simulink model "test1"  (R2022b)
settings: Solver=VariableStepAuto  StartTime=0.0  StopTime=120  RelTol=1e-3
libraries: simulink x7, simulink_extras x3, slpidlib x1
settings Model: Creator=littl  LastModifiedBy=littl

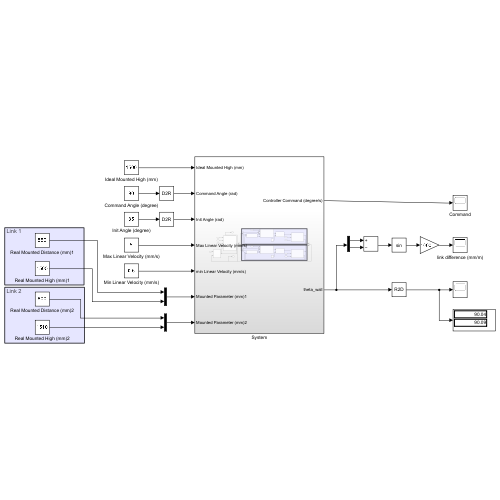
[thumbnail: Simulink's stored preview of the top-level diagram]
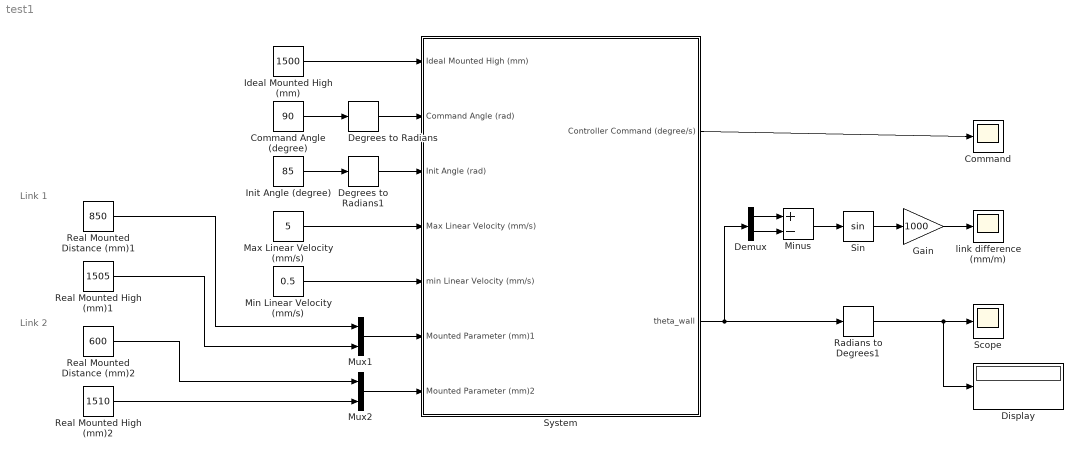
== system test1 ==
  note: Link 1
  note: Link 2
  Command : Scope
  Command Angle (degree) : Constant  Value=90
  Degrees to Radians : simulink_extras/Transformations/Degrees to Radians
  Degrees to Radians1 : simulink_extras/Transformations/Degrees to Radians
  Demux : Demux  Outputs=2
  Display : Display
  Gain : Gain  Gain=1000
  Ideal Mounted High (mm) : Constant  Value=1500
  Init Angle (degree) : Constant  Value=85
  Max Linear Velocity (mm/s) : Constant  Value=5
  Min Linear Velocity (mm/s) : Constant  Value=0.5
  Minus : Sum  Inputs=+-
  Mux1 : Mux  Inputs=2
  Mux2 : Mux  Inputs=2
  Radians to Degrees1 : simulink_extras/Transformations/Radians to Degrees
  Real Mounted Distance (mm)1 : Constant  Value=850
  Real Mounted Distance (mm)2 : Constant  Value=600
  Real Mounted High (mm)1 : Constant  Value=1505
  Real Mounted High (mm)2 : Constant  Value=1510
  Scope : Scope
  Sin : Trigonometry
  System : Subsystem
  link difference (mm/m) : Scope
  wires:
  Command Angle (degree)/1 -> Degrees to Radians/1
  Init Angle (degree)/1 -> Degrees to Radians1/1
  Minus/1 -> Sin/1
  Ideal Mounted High (mm)/1 -> System/1(Ideal Mounted High (mm))
  Degrees to Radians/1 -> System/2(Command Angle (rad))
  Degrees to Radians1/1 -> System/3(Init Angle (rad))
  System/1(Controller Command (degree/s)) -> Command/1
  Max Linear Velocity (mm/s)/1 -> System/4(Max Linear Velocity (mm/s))
  Min Linear Velocity (mm/s)/1 -> System/5(min Linear Velocity (mm/s))
  Demux/2 -> Minus/2
  Demux/1 -> Minus/1
  Radians to Degrees1/1 -> Display/1, Scope/1
  Sin/1 -> Gain/1
  Gain/1 -> link difference (mm/m)/1
  System/2(theta_wall) -> Radians to Degrees1/1, Demux/1
  Mux1/1 -> System/6(Mounted Parameter (mm)1)
  Real Mounted Distance (mm)1/1 -> Mux1/1
  Real Mounted High (mm)1/1 -> Mux1/2
  Real Mounted Distance (mm)2/1 -> Mux2/1
  Real Mounted High (mm)2/1 -> Mux2/2
  Mux2/1 -> System/7(Mounted Parameter (mm)2)

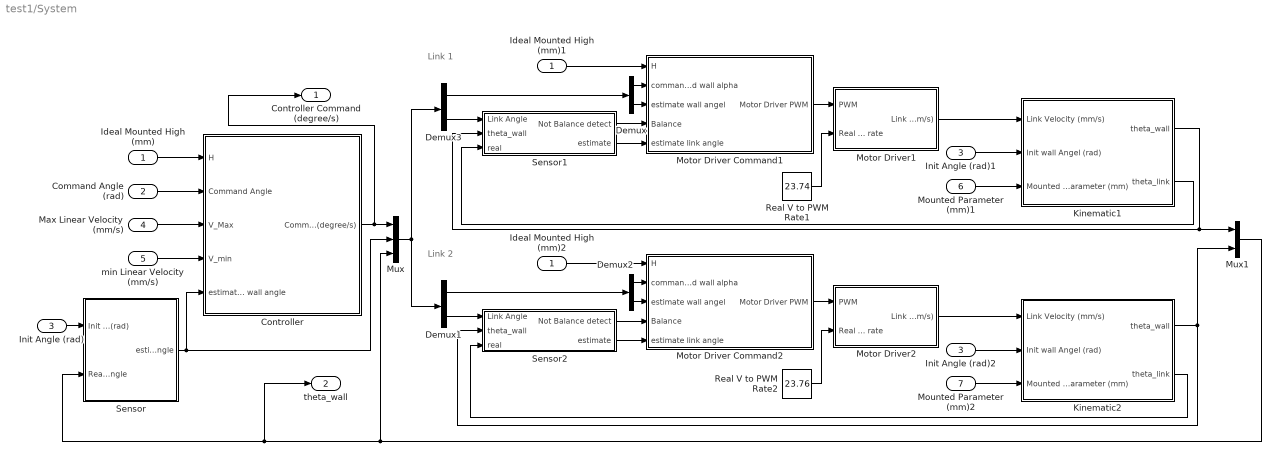
== system test1/System ==
  note: Link 1
  note: Link 2
  Ideal Mounted High (mm) : Inport
  Command Angle (rad) : Inport  Port=2
  Init Angle (rad) : Inport  Port=3
  Max Linear Velocity (mm/s) : Inport  Port=4
  min Linear Velocity (mm/s) : Inport  Port=5
  Mounted Parameter (mm)1 : Inport  Port=6
  Mounted Parameter (mm)2 : Inport  Port=7
  Controller : Subsystem
  Demux{,1..3} (4 alike) : Demux  Outputs=2
  Ideal Mounted High (mm)1 : InportShadow
  Ideal Mounted High (mm)2 : InportShadow
  Init Angle (rad)1 : InportShadow  Port=3
  Init Angle (rad)2 : InportShadow  Port=3
  Kinematic1 : Subsystem
  Kinematic2 : Subsystem
  Motor Driver Command1 : Subsystem
  Motor Driver Command2 : Subsystem
  Motor Driver1 : Subsystem
  Motor Driver2 : Subsystem
  Mux : Mux  Inputs=3
  Mux1 : Mux  Inputs=2
  Real V to PWM Rate1 : Constant  Value=23.74
  Real V to PWM Rate2 : Constant  Value=23.76
  Sensor : Subsystem
  Sensor1 : Subsystem
  Sensor2 : Subsystem
  Controller Command (degree/s) : Outport
  theta_wall : Outport  Port=2
  wires:
  min Linear Velocity (mm/s)/1 -> Controller/4(V_min)
  Motor Driver Command2/1(Motor Driver PWM) -> Motor Driver2/1(PWM)
  Real V to PWM Rate1/1 -> Motor Driver1/2(Real V to PWM rate)
  Max Linear Velocity (mm/s)/1 -> Controller/3(V_Max)
  Kinematic2/1(theta_wall) -> Mux1/2, Sensor2/2(theta_wall)
  Command Angle (rad)/1 -> Controller/2(Command Angle)
  Mounted Parameter (mm)2/1 -> Kinematic2/3(Mounted Parameter (mm))
  Real V to PWM Rate2/1 -> Motor Driver2/2(Real V to PWM rate)
  Controller/1(Command alpha (degree/s)) -> Controller Command (degree/s)/1, Mux/1
  Mounted Parameter (mm)1/1 -> Kinematic1/3(Mounted Parameter (mm))
  Motor Driver Command1/1(Motor Driver PWM) -> Motor Driver1/1(PWM)
  Motor Driver1/1(Link Velocity (mm/s)) -> Kinematic1/1(Link Velocity (mm/s))
  Motor Driver2/1(Link Velocity (mm/s)) -> Kinematic2/1(Link Velocity (mm/s))
  Ideal Mounted High (mm)2/1 -> Motor Driver Command2/1(H)
  Ideal Mounted High (mm)/1 -> Controller/1(H)
  Init Angle (rad)1/1 -> Kinematic1/2(Init wall Angel (rad))
  Init Angle (rad)2/1 -> Kinematic2/2(Init wall Angel (rad))
  Mux/1 -> Demux3/1, Demux1/1
  Sensor/1(estimate wall angle) -> Controller/5(estimate wall angle), Mux/2
  Init Angle (rad)/1 -> Sensor/1(Init Angle (rad))
  Kinematic1/1(theta_wall) -> Mux1/1, Sensor1/2(theta_wall)
  Mux1/1 -> Mux/3, theta_wall/1, Sensor/2(Real Angle)
  Demux2/1 -> Motor Driver Command2/2(command wall alpha)
  Demux2/2 -> Motor Driver Command2/3(estimate wall angel)
  Demux1/1 -> Demux2/1
  Demux/1 -> Motor Driver Command1/2(command wall alpha)
  Demux/2 -> Motor Driver Command1/3(estimate wall angel)
  Ideal Mounted High (mm)1/1 -> Motor Driver Command1/1(H)
  Demux3/1 -> Demux/1
  Demux3/2 -> Sensor1/1(Link Angle)
  Kinematic1/2(theta_link) -> Sensor1/3(real)
  Sensor1/1(Not Balance detect) -> Motor Driver Command1/4(Balance)
  Sensor1/2(estimate) -> Motor Driver Command1/5(estimate link angle)
  Demux1/2 -> Sensor2/1(Link Angle)
  Kinematic2/2(theta_link) -> Sensor2/3(real)
  Sensor2/1(Not Balance detect) -> Motor Driver Command2/4(Balance)
  Sensor2/2(estimate) -> Motor Driver Command2/5(estimate link angle)

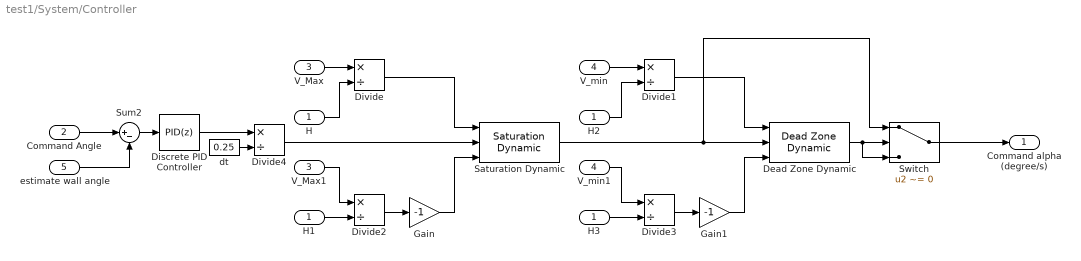
== system test1/System/Controller ==
  H : Inport
  Command Angle : Inport  Port=2
  V_Max : Inport  Port=3
  V_min : Inport  Port=4
  estimate wall angle : Inport  Port=5
  Dead Zone Dynamic : simulink/Discontinuities/Dead Zone Dynamic
  Discrete PID Controller : slpidlib/PID Controller  Controller=PID  Form=Parallel  TimeDomain=Discrete-time  UseExternalTs=off  SampleTime=0.25  IntegratorMethod=Forward Euler  FilterMethod=Forward Euler  ControllerParametersSource=internal  P=0.13  I=3e-5  UseKiTs=off  D=0.1  N=100  UseFilter=off  TunerSelectOption=Transfer Function Based (PID Tuner App)  ZeroCross=off  InitialConditionSource=internal  InitialConditionForIntegrator=0  InitialConditionForFilter=0  DifferentiatorICPrevScaledInput=0  ExternalReset=none  TrackingMode=off  Kt=1  LimitOutput=off  SatLimitsSource=internal  UpperSaturationLimit=inf  LowerSaturationLimit=-inf  LinearizeAsGain=off  AntiWindupMode=none  Kb=1  LimitIntegrator=off  UpperIntegratorSaturationLimit=inf  LowerIntegratorSaturationLimit=-inf  RndMeth=Ceiling  PGainOutDataTypeStr=Inherit: Inherit via back propagation  PProdOutDataTypeStr=Inherit: Inherit via back propagation  POutMin=[]  POutMax=[]  IOutMin=[]  IOutMax=[]  DOutMin=[]  DOutMax=[]  NOutMin=[]  NOutMax=[]  SumOutMin=[]  SumOutMax=[]  SaturationOutMin=[]  SaturationOutMax=[]  PParamMin=[]  PParamMax=[]  IParamMin=[]  IParamMax=[]  DParamMin=[]  DParamMax=[]  NParamMin=[]  NParamMax=[]  KbParamMin=[]  KbParamMax=[]  KtParamMin=[]  KtParamMax=[]  KbOutMin=[]  KbOutMax=[]  KtOutMin=[]  KtOutMax=[]  IntegratorOutMin=[]  IntegratorOutMax=[]  FilterOutMin=[]  FilterOutMax=[]  SumI1OutMin=[]  SumI1OutMax=[]  SumI2OutMin=[]  SumI2OutMax=[]  SumI3OutMin=[]  SumI3OutMax=[]  SumI4OutMin=[]  SumI4OutMax=[]  SumDOutMin=[]  SumDOutMax=[]  DifferentiatorOutMin=[]  DifferentiatorOutMax=[]  FilterDiffOutCoefMin=[]  FilterDiffOutCoefMax=[]  ReciprocalOutMin=[]  ReciprocalOutMax=[]  SumDenOutMin=[]  SumDenOutMax=[]  SumNumOutMin=[]  SumNumOutMax=[]  DivideOutMin=[]  DivideOutMax=[]  UdiffTsProdOutMin=[]  UdiffTsProdOutMax=[]  NTsProdOutMin=[]  NTsProdOutMax=[]  UintegralTsProdOutMin=[]  UintegralTsProdOutMax=[]  UngainTsProdOutMin=[]  UngainTsProdOutMax=[]  ClampingZeroOutDataTypeStr=Inherit: Inherit via back propagation  ClampingZeroOutMin=[]  ClampingZeroOutMax=[]  FilterDenConstantOutDataTypeStr=Inherit: Inherit via back propagation  FilterDenConstantOutMin=[]  FilterDenConstantOutMax=[]  PCopyOutDataTypeStr=Inherit: Inherit via back propagation  PCopyOutMin=[]  PCopyOutMax=[]  NCopyOutDataTypeStr=Inherit: Inherit via back propagation  NCopyOutMin=[]  NCopyOutMax=[]  IntegratorContinuousStateAttributes=''  IntegratorStateMustResolveToSignalObject=off  IntegratorRTWStateStorageClass=Auto  FilterContinuousStateAttributes=''  FilterStateMustResolveToSignalObject=off  FilterRTWStateStorageClass=Auto  ParallelPVariant=InternalParameters  IdealPVariant=Disabled  IVariant=InternalParameters  DVariant=InternalParameters  IntegratorVariant=Discrete  SatVariant=Disabled  AWVariant=Passthrough  PCopyVariant=Disabled  TRVariant=Disabled  FdbkBlocksVariant=Forward  IdealPFdbkVariant=Disabled  SatFdbkVariant=Disabled  DerivativeFilterVariant=Differentiator  NVariant=Passthrough  NCopyVariant=Disabled_SignalSpec  FilterICVariant=InternalICsDifferentiator  IntegratorICVariant=InternalICs  ExternalResetVariant=Disabled  TRSumVariant=Passthrough  SumFdbkVariant=Disabled  SumVariant=Sum_PID  TsampFilterVariant=InternalTs  TsampNgainVariant=Passthrough  TsampIntegralVariant=Passthrough  ExternalSaturationOutDataTypeStr=Inherit: Same as second input
      settings: LibrarySourceBlock=simulink/Discrete/Discrete PID Controller
  Divide{,1..4} (5 alike) : Product  Inputs=*/
  Gain : Gain  Gain=-1
  Gain1 : Gain  Gain=-1
  H1 : InportShadow
  H2 : InportShadow
  H3 : InportShadow
  Saturation Dynamic : simulink/Discontinuities/Saturation Dynamic  OutMin=[]  OutMax=[]  OutDataTypeStr=Inherit: Same as second input  OutDataType=fixdt(1, 16)  OutScaling=2^-10  DoSatur=off
  Sum2 : Sum  Inputs=|+-
  Switch : Switch  Criteria=u2 ~= 0  SaturateOnIntegerOverflow=off  InputSameDT=off
  V_Max1 : InportShadow  Port=3
  V_min1 : InportShadow  Port=4
  dt : Constant  Value=0.25
  Command alpha (degree/s) : Outport
  wires:
  Sum2/1 -> Discrete PID Controller/1
  Command Angle/1 -> Sum2/1
  estimate wall angle/1 -> Sum2/2
  Divide2/1 -> Gain/1
  H1/1 -> Divide2/2
  V_Max/1 -> Divide/1
  H/1 -> Divide/2
  Gain/1 -> Saturation Dynamic/3
  Divide/1 -> Saturation Dynamic/1
  H3/1 -> Divide3/2
  V_min1/1 -> Divide3/1
  H2/1 -> Divide1/2
  V_min/1 -> Divide1/1
  Divide1/1 -> Dead Zone Dynamic/1
  Divide3/1 -> Gain1/1
  Gain1/1 -> Dead Zone Dynamic/3
  V_Max1/1 -> Divide2/1
  Saturation Dynamic/1 -> Switch/1, Dead Zone Dynamic/2
  Dead Zone Dynamic/1 -> Switch/3, Switch/2
  Switch/1 -> Command alpha (degree/s)/1
  Discrete PID Controller/1 -> Divide4/1
  Divide4/1 -> Saturation Dynamic/2
  dt/1 -> Divide4/2

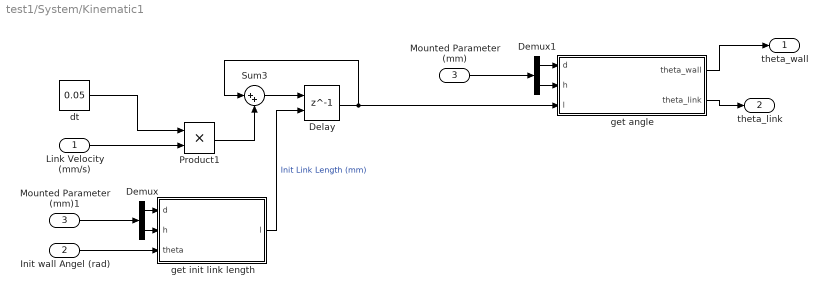
== system test1/System/Kinematic1 ==
  Link Velocity (mm/s) : Inport
  Init wall Angel (rad) : Inport  Port=2
  Mounted Parameter (mm) : Inport  Port=3
  Delay : Delay  DelayLength=1  InitialConditionSource=Input port  SampleTime=0.125
      settings: InputPortMap=u0,p4
  Demux : Demux  Outputs=2
  Demux1 : Demux  Outputs=2
  Mounted Parameter (mm)1 : InportShadow  Port=3
  Product1 : Product
  Sum3 : Sum  Inputs=|++
  dt : Constant  Value=0.05
  get angle : MATLAB Function  TreatAsAtomicUnit=on
  get init link length : MATLAB Function  TreatAsAtomicUnit=on
  theta_wall : Outport
  theta_link : Outport  Port=2
  wires:
  get angle/2(theta_link) -> theta_link/1
  get angle/1(theta_wall) -> theta_wall/1
  Sum3/1 -> Delay/1
  Delay/1 -> Sum3/1, get angle/3(l)
  Product1/1 -> Sum3/2
  get init link length/1(l) -> Delay/2  "Init Link Length (mm)"
  Init wall Angel (rad)/1 -> get init link length/3(theta)
  Link Velocity (mm/s)/1 -> Product1/2
  dt/1 -> Product1/1
  Demux/1 -> get init link length/1(d)
  Mounted Parameter (mm)1/1 -> Demux/1
  Demux/2 -> get init link length/2(h)
  Demux1/1 -> get angle/1(d)
  Demux1/2 -> get angle/2(h)
  Mounted Parameter (mm)/1 -> Demux1/1

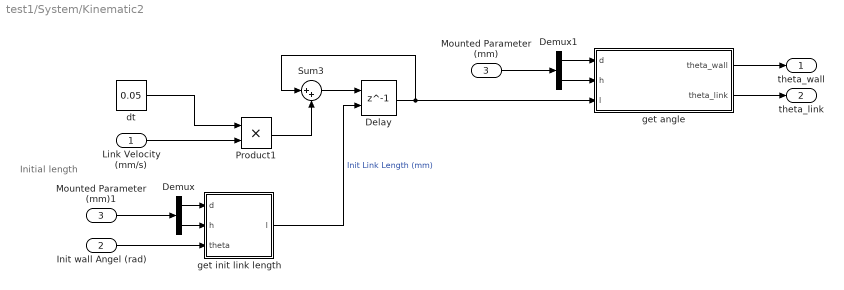
== system test1/System/Kinematic2 ==
  note: Initial length
  Link Velocity (mm/s) : Inport
  Init wall Angel (rad) : Inport  Port=2
  Mounted Parameter (mm) : Inport  Port=3
  Delay : Delay  DelayLength=1  InitialConditionSource=Input port  SampleTime=0.125
      settings: InputPortMap=u0,p4
  Demux : Demux  Outputs=2
  Demux1 : Demux  Outputs=2
  Mounted Parameter (mm)1 : InportShadow  Port=3
  Product1 : Product
  Sum3 : Sum  Inputs=|++
  dt : Constant  Value=0.05
  get angle : MATLAB Function  TreatAsAtomicUnit=on
  get init link length : MATLAB Function  TreatAsAtomicUnit=on
  theta_wall : Outport
  theta_link : Outport  Port=2
  wires:
  get angle/2(theta_link) -> theta_link/1
  get angle/1(theta_wall) -> theta_wall/1
  Sum3/1 -> Delay/1
  Delay/1 -> Sum3/1, get angle/3(l)
  Product1/1 -> Sum3/2
  get init link length/1(l) -> Delay/2  "Init Link Length (mm)"
  Init wall Angel (rad)/1 -> get init link length/3(theta)
  Link Velocity (mm/s)/1 -> Product1/2
  dt/1 -> Product1/1
  Demux/1 -> get init link length/1(d)
  Demux/2 -> get init link length/2(h)
  Mounted Parameter (mm)1/1 -> Demux/1
  Mounted Parameter (mm)/1 -> Demux1/1
  Demux1/1 -> get angle/1(d)
  Demux1/2 -> get angle/2(h)

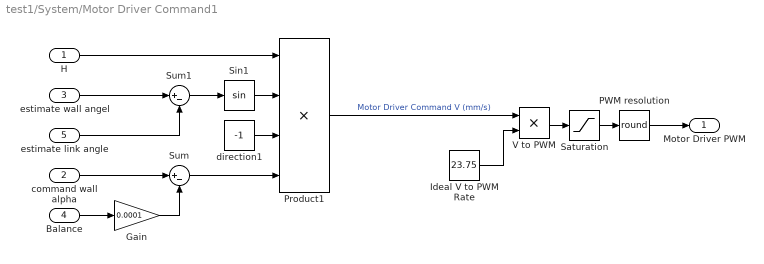
== system test1/System/Motor Driver Command1 ==
  H : Inport
  command wall alpha : Inport  Port=2
  estimate wall angel : Inport  Port=3
  Balance : Inport  Port=4
  estimate link angle : Inport  Port=5
  Gain : Gain  Gain=0.0001
  Ideal V to PWM Rate : Constant  Value=23.75
  PWM resolution : Rounding  Operator=round
  Product1 : Product  Inputs=4
  Saturation : Saturate  UpperLimit=255  LowerLimit=-255
  Sin1 : Trigonometry
  Sum : Sum  Inputs=|+-
  Sum1 : Sum  Inputs=|+-
  V to PWM : Product
  direction1 : Constant  Value=-1
  Motor Driver PWM : Outport
  wires:
  Ideal V to PWM Rate/1 -> V to PWM/2
  V to PWM/1 -> Saturation/1
  Saturation/1 -> PWM resolution/1
  PWM resolution/1 -> Motor Driver PWM/1
  Balance/1 -> Gain/1
  Sin1/1 -> Product1/2
  estimate link angle/1 -> Sum1/2
  Gain/1 -> Sum/2
  command wall alpha/1 -> Sum/1
  estimate wall angel/1 -> Sum1/1
  H/1 -> Product1/1
  Sum/1 -> Product1/4
  direction1/1 -> Product1/3
  Sum1/1 -> Sin1/1
  Product1/1 -> V to PWM/1  "Motor Driver Command V (mm/s)"

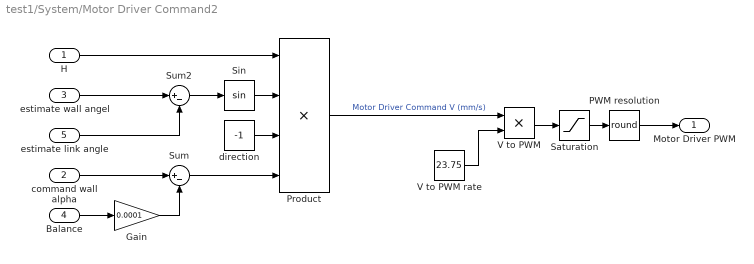
== system test1/System/Motor Driver Command2 ==
  H : Inport
  command wall alpha : Inport  Port=2
  estimate wall angel : Inport  Port=3
  Balance : Inport  Port=4
  estimate link angle : Inport  Port=5
  Gain : Gain  Gain=0.0001
  PWM resolution : Rounding  Operator=round
  Product : Product  Inputs=4
  Saturation : Saturate  UpperLimit=255  LowerLimit=-255
  Sin : Trigonometry
  Sum : Sum  Inputs=|+-
  Sum2 : Sum  Inputs=|+-
  V to PWM : Product
  V to PWM rate : Constant  Value=23.75
  direction : Constant  Value=-1
  Motor Driver PWM : Outport
  wires:
  Sum2/1 -> Sin/1
  estimate link angle/1 -> Sum2/2
  Saturation/1 -> PWM resolution/1
  Product/1 -> V to PWM/1  "Motor Driver Command V (mm/s)"
  V to PWM rate/1 -> V to PWM/2
  PWM resolution/1 -> Motor Driver PWM/1
  V to PWM/1 -> Saturation/1
  estimate wall angel/1 -> Sum2/1
  Balance/1 -> Gain/1
  command wall alpha/1 -> Sum/1
  Gain/1 -> Sum/2
  H/1 -> Product/1
  Sin/1 -> Product/2
  direction/1 -> Product/3
  Sum/1 -> Product/4

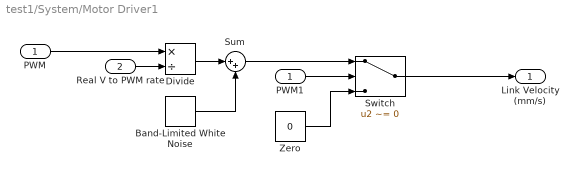
== system test1/System/Motor Driver1 ==
  PWM : Inport
  Real V to PWM rate : Inport  Port=2
  Band-Limited White Noise : simulink/Sources/Band-Limited White Noise  Cov=[0.001]  Ts=0.05  seed=[23341]
  Divide : Product  Inputs=*/
  PWM1 : InportShadow
  Sum : Sum  Inputs=|++
  Switch : Switch  Criteria=u2 ~= 0  SaturateOnIntegerOverflow=off  InputSameDT=off
  Zero : Constant  Value=0  OutDataTypeStr=Inherit: Inherit via back propagation
  Link Velocity (mm/s) : Outport
  wires:
  Switch/1 -> Link Velocity (mm/s)/1
  Real V to PWM rate/1 -> Divide/2
  PWM/1 -> Divide/1
  Divide/1 -> Sum/1
  Band-Limited White Noise/1 -> Sum/2
  Sum/1 -> Switch/1
  PWM1/1 -> Switch/2
  Zero/1 -> Switch/3

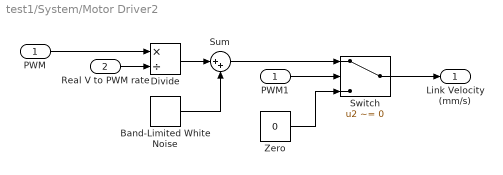
== system test1/System/Motor Driver2 ==
  PWM : Inport
  Real V to PWM rate : Inport  Port=2
  Band-Limited White Noise : simulink/Sources/Band-Limited White Noise  Cov=[0.001]  Ts=0.05  seed=[23341]
  Divide : Product  Inputs=*/
  PWM1 : InportShadow
  Sum : Sum  Inputs=|++
  Switch : Switch  Criteria=u2 ~= 0  SaturateOnIntegerOverflow=off  InputSameDT=off
  Zero : Constant  Value=0  OutDataTypeStr=Inherit: Inherit via back propagation
  Link Velocity (mm/s) : Outport
  wires:
  Switch/1 -> Link Velocity (mm/s)/1
  Real V to PWM rate/1 -> Divide/2
  PWM/1 -> Divide/1
  Divide/1 -> Sum/1
  Band-Limited White Noise/1 -> Sum/2
  Sum/1 -> Switch/1
  PWM1/1 -> Switch/2
  Zero/1 -> Switch/3

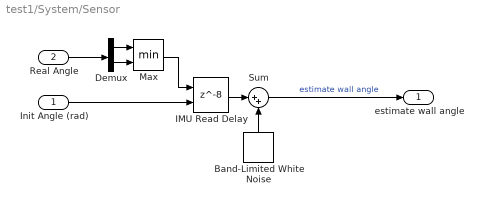
== system test1/System/Sensor ==
  Init Angle (rad) : Inport
  Real Angle : Inport  Port=2
  Band-Limited White Noise : simulink/Sources/Band-Limited White Noise  Cov=1e-10  Ts=0.05  seed=[23341]
  Demux : Demux  Outputs=2
  IMU Read Delay : Delay  DelayLength=8  InitialConditionSource=Input port  SampleTime=0.25
      settings: InputPortMap=u0,p4
  Max : MinMax  Inputs=2
  Sum : Sum  Inputs=|++
  estimate wall angle : Outport
  wires:
  Init Angle (rad)/1 -> IMU Read Delay/2
  IMU Read Delay/1 -> Sum/1
  Band-Limited White Noise/1 -> Sum/2
  Sum/1 -> estimate wall angle/1  "estimate wall angle"
  Real Angle/1 -> Demux/1
  Demux/2 -> Max/2
  Demux/1 -> Max/1
  Max/1 -> IMU Read Delay/1

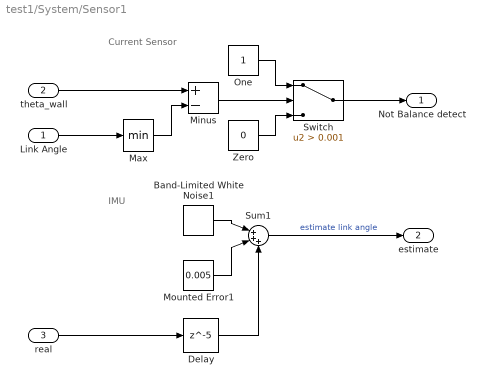
== system test1/System/Sensor1 ==
  note: IMU
  note: Current Sensor
  Link Angle : Inport
  theta_wall : Inport  Port=2
  real : Inport  Port=3
  Band-Limited White Noise1 : simulink/Sources/Band-Limited White Noise  Cov=1e-10  Ts=0.05  seed=[23341]
  Delay : Delay  DelayLength=5  SampleTime=0.1
  Max : MinMax
  Minus : Sum  Inputs=+-
  Mounted Error1 : Constant  Value=0.005
  One : Constant  OutDataTypeStr=Inherit: Inherit via back propagation
  Sum1 : Sum  Inputs=|+++
  Switch : Switch  Criteria=u2 > Threshold  Threshold=0.001  SaturateOnIntegerOverflow=off  InputSameDT=off
  Zero : Constant  Value=0  OutDataTypeStr=Inherit: Inherit via back propagation
  Not Balance detect : Outport
  estimate : Outport  Port=2
  wires:
  Switch/1 -> Not Balance detect/1
  Zero/1 -> Switch/3
  One/1 -> Switch/1
  Minus/1 -> Switch/2
  Max/1 -> Minus/2
  theta_wall/1 -> Minus/1
  Link Angle/1 -> Max/1
  Delay/1 -> Sum1/3
  real/1 -> Delay/1
  Mounted Error1/1 -> Sum1/2
  Sum1/1 -> estimate/1  "estimate link angle"
  Band-Limited White Noise1/1 -> Sum1/1

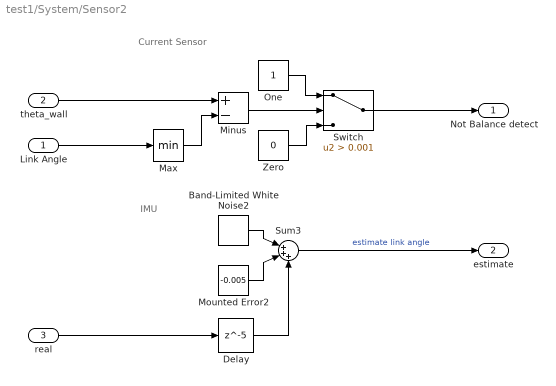
== system test1/System/Sensor2 ==
  note: IMU
  note: Current Sensor
  Link Angle : Inport
  theta_wall : Inport  Port=2
  real : Inport  Port=3
  Band-Limited White Noise2 : simulink/Sources/Band-Limited White Noise  Cov=1e-10  Ts=0.05  seed=[23341]
  Delay : Delay  DelayLength=5  SampleTime=0.1
  Max : MinMax
  Minus : Sum  Inputs=+-
  Mounted Error2 : Constant  Value=-0.005
  One : Constant  OutDataTypeStr=Inherit: Inherit via back propagation
  Sum3 : Sum  Inputs=|+++
  Switch : Switch  Criteria=u2 > Threshold  Threshold=0.001  SaturateOnIntegerOverflow=off  InputSameDT=off
  Zero : Constant  Value=0  OutDataTypeStr=Inherit: Inherit via back propagation
  Not Balance detect : Outport
  estimate : Outport  Port=2
  wires:
  Switch/1 -> Not Balance detect/1
  Zero/1 -> Switch/3
  One/1 -> Switch/1
  Minus/1 -> Switch/2
  Max/1 -> Minus/2
  theta_wall/1 -> Minus/1
  Link Angle/1 -> Max/1
  Delay/1 -> Sum3/3
  real/1 -> Delay/1
  Band-Limited White Noise2/1 -> Sum3/1
  Mounted Error2/1 -> Sum3/2
  Sum3/1 -> estimate/1  "estimate link angle"

== matlab function test1/System/Kinematic1/get init link length ==
  data: d input; h input; l output; theta input
function l = cosines(d,h,theta)
%#codegen
l = (h^2 + d^2 - 2 * h * d *cos(pi-theta))^0.5;

== matlab function test1/System/Kinematic1/get angle ==
  data: d input; h input; l input; theta_wall output; theta_link output
function [theta_wall, theta_link] = arccosines(d,h,l)
theta_link = acos((l^2+d^2-h^2)/(2*l*d));
theta_wall = pi-acos((h^2+d^2-l^2)/(2*h*d));

== matlab function test1/System/Kinematic2/get angle ==
  data: d input; h input; l input; theta_wall output; theta_link output
function [theta_wall, theta_link] = triangle(d,h,l)
theta_link = acos((l^2+d^2-h^2)/(2*l*d));
theta_wall = pi-acos((h^2+d^2-l^2)/(2*h*d));

== matlab function test1/System/Kinematic2/get init link length ==
  data: d input; h input; l output; theta input
function l = fcn(d,h,theta)
%#codegen
l = (h^2 + d^2 - 2 * h * d *cos(pi-theta))^0.5;
